simulink model "rtwdemo_configurable_sys"  (Simulink 7.6)
settings: Solver=FixedStepDiscrete  StartTime=0.0  StopTime=0.5  FixedStep=1/60  RelTol=1e-3  AbsTol=1e-6
PreLoadFcn:
  | width = 160;
undefined symbols (not defined in the file or in its folder): DiscIntNeverNeededParam
libraries: vxlib1 x2, rtwdemo_configurable_source x1
settings Model: Creator=The MathWorks Inc.  ExtModeTrigMode=oneshot  ExtModeArmWhenConnect=off  ExtModeAutoUpdateStatusClock=off
settings SolverCC: AutoInsertRateTranBlk=on
settings MATStruct: SampleTime=1/60  Offset=0  Priority=[20.0]
settings DataIOCC: LimitDataPoints=off  SaveOutput=off  SaveTime=off  SignalLoggingName=sigsOut
settings OptimizationCC: InlineParams=on  InlineInvariantSignals=on  StateBitsets=on  DataBitsets=on  UseTempVars=on  EfficientFloat2IntCast=on  EfficientMapNaN2IntZero=off  LifeSpan=1
settings DebuggingCC: CheckExecutionContextPreStartOutputMsg=on  CheckExecutionContextRuntimeOutputMsg=on  SolverPrmCheckMsg=none  InheritedTsInSrcMsg=none  IntegerOverflowMsg=none  UnconnectedInputMsg=none  UnconnectedOutputMsg=none  UnconnectedLineMsg=none  StrictBusMsg=ErrorOnBusTreatedAsVector
settings HardwareCC: ProdIntDivRoundTo=Zero  ProdEndianess=LittleEndian  ProdHWDeviceType=Generic->32-bit Embedded Processor  TargetHWDeviceType=Generic->32-bit Embedded Processor
settings ModelReferenceCC: UpdateModelReferenceTargets=IfOutOfDate
settings RTWCC: SystemTargetFile=tornado.tlc  TLCOptions=-p0 -aWarnNonSaturatedBlocks=0  GenCodeOnly=on  TemplateMakefile=tornado.tmf  Description=Tornado (VxWorks) Real-Time Target  GenerateReport=on  RTWVerbose=off  ProcessScript=tornado_make_rtw_hook  LaunchReport=on
settings CodeAppCC: ForceParamTrailComments=on
settings TornadoTargetCC: TargetFcnLib=ansi_tfl_tmw.mat  TargetFunctionLibrary=ANSI_C  UtilityFuncGeneration=Auto  ERTMultiwordTypeDef=System defined  ERTCodeCoverageTool=None  ERTMultiwordLength=256  MultiwordLength=2048  GenerateFullHeader=on  GenerateSampleERTMain=off  GenerateTestInterfaces=off  IsPILTarget=off  ModelReferenceCompliant=off  ParMdlRefBuildCompliant=on  CompOptLevelCompliant=off  IncludeMdlTerminateFcn=on  GeneratePreprocessorConditionals=Disable all  CombineOutputUpdateFcns=off  CombineSignalStateStructs=off  SuppressErrorStatus=off  ERTFirstTimeCompliant=off  IncludeFileDelimiter=Auto  ERTCustomFileBanners=off  SupportAbsoluteTime=on  LogVarNameModifier=rt_  MatFileLogging=off  MultiInstanceERTCode=off  SupportNonFinite=on  SupportComplex=on  PurelyIntegerCode=off  SupportContinuousTime=on  SupportNonInlinedSFcns=on  SupportVariableSizeSignals=off  EnableShiftOperators=on  ParenthesesLevel=Nominal  PortableWordSizes=off  ModelStepFunctionPrototypeControlCompliant=off  CPPClassGenCompliant=off  AutosarCompliant=off  CodeFormat=RealTime  StethoScope=off  DownloadToVxWorks=off  BasePriority=30  TaskStackSize=16384  ExtMode=off  ExtModeTransport=0  ExtModeStaticAlloc=off  ExtModeStaticAllocSize=1000000  ExtModeTesting=off  ExtModeMexFile=ext_comm  ExtModeIntrfLevel=Level1  RTWCAPIParams=off  RTWCAPISignals=off

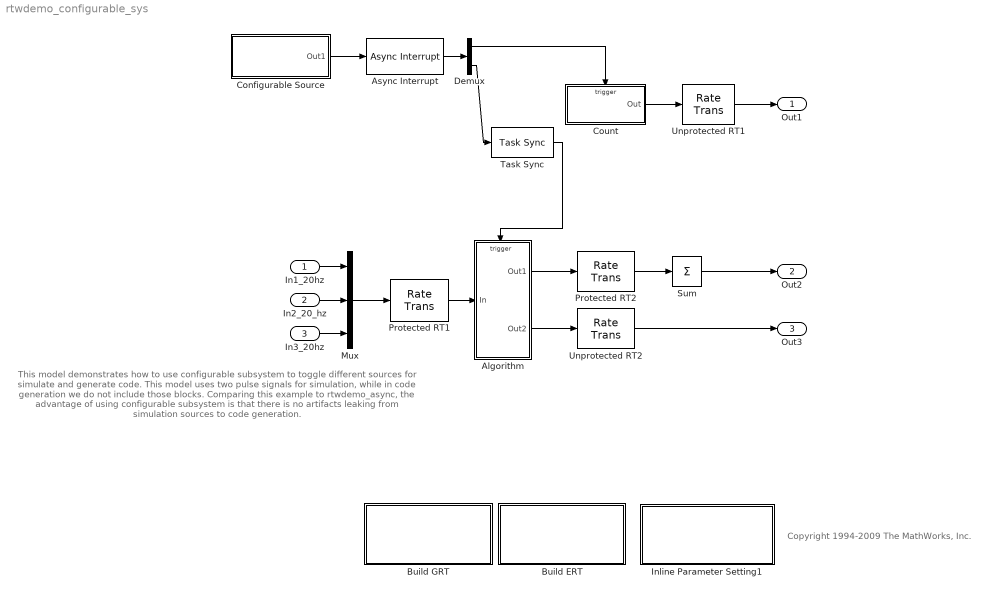
== system rtwdemo_configurable_sys ==
  note: This model demonstrates how to use configurable subsystem to toggle different sources for simulate and generate code.
      | This model uses two pulse signals for simulation, while in code generation we do not include those blocks.  Comparing
      | this example to rtwdemo_async, the advantage of using configurable subsystem is that there is no artifacts leaking
      | from simulation sources to code generation.
  note: Copyright 1994-2009 The MathWorks, Inc.
  In1_20hz : Inport  OutDataTypeStr=double  PortDimensions=20  SampleTime=1/20
  In2_20_hz : Inport  Port=2  OutDataTypeStr=double  PortDimensions=20  SampleTime=1/20
  In3_20hz : Inport  Port=3  OutDataTypeStr=double  PortDimensions=20  SampleTime=1/20
  Algorithm : Subsystem  TreatAsAtomicUnit=on  RTWFcnName=Algorithm  RTWFileName=Algorithm
      settings: RTWFcnNameOpts=User specified  RTWFileNameOpts=User specified
  Async Interrupt : vxlib1/Async Interrupt  irqnumbers=[1 2]  irqoffsets=[192 193]  irqpriorities=[10 11]  irqpreempts=[0 1]  manageowntimer=on  tickres=1/60  ticklen=32bits  showinput=on
  Build ERT : Subsystem  mask{attrib_overrides={'IncludeMdlTerminateFcn'}}
      mask prompts: attrib_overrides "List of attributes to preserve (cell of strings):"
      mask help: Enter the attributes of the configuration set that you want preserved. Otherwise, the default configuration script will override your current settings.
      settings: OpenFcn=|
      | model=bdroot;
      |                   overrides=get_param(gcb,'attrib_overrides');
      | try
      |   rtwconfiguredemo(model,'noop',false,overrides);
      |   cs = getActiveConfigSet(bdroot);
      |   set_param(cs,'TargetOS','VxWorksExample');
      |   rtwbuilddemomodel(model);
      | catch
      |   error(lasterr);
      | end
      |                           clear model overrides cs;
      mask Display:
      | disp(['Generate Code Using\n',...
      | 	  'Real-Time Workshop\n',...
      | 	  'Embedded Coder\n'...
      | 	  '(double-click)'])
  Build GRT : Subsystem  mask{attrib_overrides={}}
      mask prompts: attrib_overrides "List of attributes to preserve (cell of strings):"
      mask help: Enter the attributes of the configuration set that you want preserved. Otherwise, the default configuration script will override your current settings.
      settings: OpenFcn=|
      | model=bdroot;
      |                   overrides=get_param(gcb,'attrib_overrides');
      | try
      |   rtwconfiguredemo(model,'noop',true,overrides);
      |   cs = getActiveConfigSet(bdroot);
      |   cs.switchTarget('tornado.tlc',[]);
      |   set_param(cs,'TemplateMakefile','tornado.tmf');              rtwbuilddemomodel(model);
      | catch
      |   error(lasterr);
      | end;
      |    clear model overrides cs;
      mask Display:
      | disp(['Generate Code Using\n',...
      | 	  'Real-Time Workshop\n',...
      | 	  '(double-click)'])
  Configurable Source : Subsystem  BlockChoice=Sim Source
      mask init:
      | if rtwenvironmentmode(bdroot(gcbh))
      | 	set_param(gcbh, 'BlockChoice', 'Sim Source');
      | else
      | 	set_param(gcbh, 'BlockChoice', 'Code Gen Source');
      | end
      settings: AttributesFormatString=%<BlockChoice>  TemplateBlock=rtwdemo_configurable_source/Configurable Source  MemberBlocks=Code Gen Source,Sim Source
      mask Display: disp('Configurable Source');
  Count : Subsystem  TreatAsAtomicUnit=on  RTWFcnName=Count  RTWFileName=Count
      settings: RTWFcnNameOpts=User specified  RTWFileNameOpts=User specified
  Demux : Demux  Outputs=2
  Inline Parameter Setting1 : Subsystem
      settings: OpenFcn=m=get_param(bdroot,'name'); eval([m,'([],[],[],''compile'');']); eval([m,'([],[],[],''term'');']); clear m;
      mask Display: disp(sprintf('Display\nSimulation Time\nSample Time Colors\n(double-click)'))
  Mux : Mux  Inputs=3
  Protected RT1 : RateTransition  Deterministic=off
  Protected RT2 : RateTransition  Deterministic=off  OutPortSampleTime=1/20
  Sum : Sum  Inputs=1  SaturateOnIntegerOverflow=on  InputSameDT=on  OutDataTypeStr=Inherit: Same as first input
  Task Sync : vxlib1/Task Sync  SystemSampleTime=-1  taskname=Task0  taskpriority=50  taskstacksize=8192  parentmanaget=on  tickres=1/60  ticklen=32bits
  Unprotected RT1 : RateTransition  Integrity=off  OutPortSampleTime=1/20
  Unprotected RT2 : RateTransition  Integrity=off  OutPortSampleTime=1/20
  Out1 : Outport
  Out2 : Outport  Port=2
  Out3 : Outport  Port=3
  wires:
  Protected RT1/1 -> Algorithm/1(In)
  Mux/1 -> Protected RT1/1
  Algorithm/1(Out1) -> Protected RT2/1
  Protected RT2/1 -> Sum/1
  Sum/1 -> Out2/1
  Task Sync/1 -> Algorithm/Trigger
  Algorithm/2(Out2) -> Unprotected RT2/1
  Unprotected RT2/1 -> Out3/1
  Count/1(Out) -> Unprotected RT1/1
  Unprotected RT1/1 -> Out1/1
  In1_20hz/1 -> Mux/1
  In2_20_hz/1 -> Mux/2
  In3_20hz/1 -> Mux/3
  Async Interrupt/1 -> Demux/1
  Demux/1 -> Count/Trigger
  Demux/2 -> Task Sync/1
  Configurable Source/1(Out1) -> Async Interrupt/1

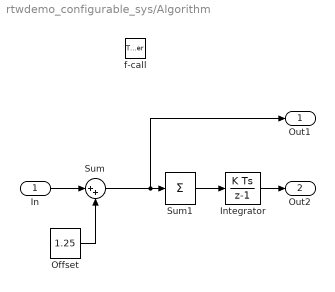
== system rtwdemo_configurable_sys/Algorithm ==
  In : Inport
  f-call : TriggerPort  TriggerType=function-call
  Integrator : DiscreteIntegrator  InitialConditionMode=State only (most efficient)  SampleTime=-1  SaturateOnIntegerOverflow=on  ICPrevOutput=DiscIntNeverNeededParam  ICPrevScaledInput=DiscIntNeverNeededParam
  Offset : Constant  Value=1.25
  Sum : Sum  Inputs=|++
  Sum1 : Sum  Inputs=1  SaturateOnIntegerOverflow=on  InputSameDT=on  OutDataTypeStr=Inherit: Same as first input
  Out1 : Outport  InitialOutput=0
  Out2 : Outport  Port=2  InitialOutput=0
  wires:
  In/1 -> Sum/1
  Sum/1 -> Sum1/1, Out1/1
  Sum1/1 -> Integrator/1
  Integrator/1 -> Out2/1
  Offset/1 -> Sum/2

== system rtwdemo_configurable_sys/Build ERT ==

== system rtwdemo_configurable_sys/Build GRT ==

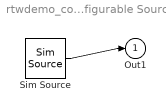
== system rtwdemo_configurable_sys/Configurable Source ==
  Sim Source : rtwdemo_configurable_source/Sim Source  SystemSampleTime=-1
  Out1 : Outport
  wires:
  Sim Source/1 -> Out1/1

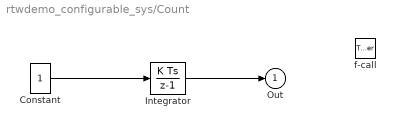
== system rtwdemo_configurable_sys/Count ==
  f-call : TriggerPort  TriggerType=function-call
  Constant : Constant
  Integrator : DiscreteIntegrator  InitialConditionMode=State only (most efficient)  SampleTime=-1  SaturateOnIntegerOverflow=on  ICPrevOutput=DiscIntNeverNeededParam  ICPrevScaledInput=DiscIntNeverNeededParam
  Out : Outport  InitialOutput=0
  wires:
  Constant/1 -> Integrator/1
  Integrator/1 -> Out/1

== system rtwdemo_configurable_sys/Inline Parameter Setting1 ==
